simulink model "Waehrungsmodelle"  (R2014a)
settings: Solver=ode1  StartTime=0.0  StopTime=100  FixedStep=1  MaxStep=1  MinStep=1  RelTol=1e-3
(part 11 of 18)

== matlab function Waehrungsmodelle/Fließendes Währungssystem/Wechselkursberechnung/MATLAB Function ==
  data: GueterpreisAuslandInEigenwaehrung output; GueterpreisAusland input; Wechselkursfaktor output; GueterKonsumImInlandVomAusland input; GueterKonsumImAuslandVomInland input; GesamterGueterKonsumImAuslandVomInlandOut output; GesamterGueterKonsumImInlandVomAuslandOut output
function [GueterpreisAuslandInEigenwaehrung, Wechselkursfaktor, GesamterGueterKonsumImAuslandVomInlandOut, GesamterGueterKonsumImInlandVomAuslandOut] ...
        = Wechselkursberechnung(GueterpreisAusland, GueterKonsumImInlandVomAusland, GueterKonsumImAuslandVomInland)
%# Untermodul zur Berechnung eines realen Wechselkurses


% Aufsummierter Güterkonsum vom Ausland mit produzierten Gütern aus dem Inland
persistent GesamterGueterKonsumImAuslandVomInland;          
        
% Aufsummierter Güterkonsum vom Inland mit produzierten Gütern aus dem Ausland
persistent GesamterGueterKonsumImInlandVomAusland;    

% GesamterGueterKonsumImAuslandVomInland Initial
if isempty(GesamterGueterKonsumImAuslandVomInland)
   GesamterGueterKonsumImAuslandVomInland = 1;
end

% GueterKonsumImInlandVomAusland Initial
if isempty(GesamterGueterKonsumImInlandVomAusland)
   GesamterGueterKonsumImInlandVomAusland = 1;
end

GesamterGueterKonsumImAuslandVomInland = GesamterGueterKonsumImAuslandVomInland + GueterKonsumImAuslandVomInland;
GesamterGueterKonsumImInlandVomAusland = GesamterGueterKonsumImInlandVomAusland + GueterKonsumImInlandVomAusland;
   
% Berechnung eines realen Wechselkurses
Wechselkursfaktor =  GesamterGueterKonsumImInlandVomAusland / GesamterGueterKonsumImAuslandVomInland;

% Güterpreis der importierten Waren in Inländischer Währung
GueterpreisAuslandInEigenwaehrung = GueterpreisAusland * Wechselkursfaktor;

% Zustandswerte ausgeben
GesamterGueterKonsumImAuslandVomInlandOut = GesamterGueterKonsumImAuslandVomInland;
GesamterGueterKonsumImInlandVomAuslandOut = GesamterGueterKonsumImInlandVomAusland;

== matlab function Waehrungsmodelle/Währungssystem5/Haushalte/MATLAB Function ==
  data: Erwerbsfaehige input; GueterkonsumInland output; ArbeitsplaetzeDienstleistungen input; ArbeitsplaetzeUnternehmen input; NeueKreditvergabeInland input; KreditrueckzahlungInland input; GueterAngebotInland input; Arbeitslohn input; GueterpreisInland input; FinanzierungArbeitslosigkeit output; Spareinlagen output; KreditbedarfInland output; ArbeiterUnternehmen output; GueterVorratHaushalte output; GueterangebotsqualitaetOut output; Arbeitslosenquote output; GueterpreisAusland input; GueterkonsumAusland output; KreditbedarfAusland output; NeueKreditvergabeAusland input; KreditrueckzahlungAusland input; GueterAngebotAusland input; KreditZinssatzInland input; KreditZinssatzAusland input
function [GueterkonsumInland, FinanzierungArbeitslosigkeit, Spareinlagen, KreditbedarfInland, ...
              ArbeiterUnternehmen, GueterVorratHaushalte, GueterangebotsqualitaetOut, ...
              Arbeitslosenquote, GueterkonsumAusland, KreditbedarfAusland] = ...
    Haushalte(Erwerbsfaehige, ArbeitsplaetzeDienstleistungen, ArbeitsplaetzeUnternehmen, ...
            NeueKreditvergabeInland, KreditrueckzahlungInland, GueterAngebotInland, Arbeitslohn, ...
            GueterpreisInland, GueterpreisAusland, NeueKreditvergabeAusland, ...
            KreditrueckzahlungAusland, GueterAngebotAusland, KreditZinssatzInland, KreditZinssatzAusland)
 %# Submodul zur Berechnung der Abläufe bzgl. der Haushalte
 
% Es wird eine Gütereinheit pro Zeiteinheit und Erwerbsfaehiger
% verbraucht;
persistent GueterVorrat;

% Angebotsqualität der Güter [0 - 1]
% Werden weniger Güter angeboten als benötigt oder ist die Anzahl der 
% benötigten Güter nicht mehr bezahlbar sinkt die Qualität
persistent Gueterangebotsqualitaet;

    % Anfangsvorrat
    if isempty(GueterVorrat)
       GueterVorrat = 100;
    end 
    
    if isempty(Gueterangebotsqualitaet)
       Gueterangebotsqualitaet = 1;
    end     
    
    % Beschäftigte bei Öffentlichen Dienstleistungen bekommen 80 % vom
    % Lohnniveau der Unternehmen
    Dienstleistungslohnfaktor = 0.8;
    
    % Arbeitslose bekommen vom Staat 50% des Lohnnivaus
    Arbeitslosenlohnfaktor = 0.5;    
    
    % Maximale Vorratszeit
    MaximaleVorratszeit = 4;
    
    % Der maximale Vorrat gilt für 4 Zeiteinheiten
    MaximalerVorrat = Erwerbsfaehige * MaximaleVorratszeit; 
    
    
    % Gueterverbrauch pro Zeiteinheit
    GueterVorrat = GueterVorrat -  Erwerbsfaehige;    

    if GueterVorrat <= 0
         % Sind weniger Vorräte als fuer eine Zeiteinheit vorhanden, 
         % sinkt die Güterqualität
        Gueterangebotsqualitaet = Gueterangebotsqualitaet - 0.1;
        Gueterangebotsqualitaet = max(Gueterangebotsqualitaet, 0);
    else 
         % Sind mehr Vorräte als fuer eine Zeiteinheit vorhanden, 
         % steigt die Güterqualität        
        Gueterangebotsqualitaet = Gueterangebotsqualitaet + 0.1;
        Gueterangebotsqualitaet = min(Gueterangebotsqualitaet, 1);        
    end       
    
    GueterangebotsqualitaetOut = Gueterangebotsqualitaet;  
    
    % Es können maximal die vergleibenden Erwerbsfähigen oder der
    % notwendige Arbeiterbedarf eingesetzt werden
    ArbeiterUnternehmen = Erwerbsfaehige - ArbeitsplaetzeDienstleistungen;
    
    % die Arbeitslosen sind alle Erwerbsfähigen, welche keinen Arbeitsplatz
    % haben
    Arbeitslose = Erwerbsfaehige - (ArbeitsplaetzeUnternehmen + ArbeitsplaetzeDienstleistungen );
    % Arbeitslosenquote [0 - 1]
    % Auf Grund von Rundungen kann die Arbeitslosenquote min. 0 sein.
    Arbeitslosenquote = max(0, Arbeitslose / Erwerbsfaehige);
    
   
    
    % Einkommensberechnung für die Arbeitsplätze bei Unternehmen
    EinkommenUnternehmen = ArbeitsplaetzeUnternehmen * Arbeitslohn ;
    
    % Einkommensberechnung für die Arbeitsplätze bei Öffentlichen Dienstleistungen
    EinkommenDienstleistungen = ArbeitsplaetzeDienstleistungen * Arbeitslohn * Dienstleistungslohnfaktor;
    
    % Finanzierungsbedarf fuer Arbeitslosigkeit
    EinkommenArbeitslosigkeit = Arbeitslose * Arbeitslohn * Arbeitslosenlohnfaktor;
    FinanzierungArbeitslosigkeit = EinkommenArbeitslosigkeit;
    
    % Berechnung des Gesamteinkommens
    Gesamteinkommen = EinkommenUnternehmen + EinkommenDienstleistungen + EinkommenArbeitslosigkeit;           
        
    % Genehmigung der letzten Kreditanfrage
    Gesamteinkommen = Gesamteinkommen + NeueKreditvergabeInland + NeueKreditvergabeAusland;   
    
    % Rückzahlung der offenen Kreditrate
    Gesamteinkommen = Gesamteinkommen - KreditrueckzahlungInland - KreditrueckzahlungAusland;    
    
    % Prüfen welche Güter die günstigeren sind (Inlandsgüter oder
    % Auslandsgüter)
    if GueterpreisInland <= GueterpreisAusland
        % Wenn die Güter im Inland günstiger sind
        
        % Güter nachkaufen solange das Geld reicht oder das Vorratsmaximum erreicht
        % wurde, in Abhängigkeit des Güterangebots
        MoeglicheGueternachfrage = floor(Gesamteinkommen / GueterpreisInland);      
        % Die kleinste Gueternachfrage ist immer 50% des normalen
        % Verbrauchs der Güter
        GueterkonsumInland = max(0, min(MoeglicheGueternachfrage, GueterAngebotInland));

        % Wenn genug Güter auf Vorrat Komsum auf 50% senken
        if GueterVorrat > MaximalerVorrat
            GueterkonsumInland = GueterkonsumInland / 2;    
        end

        GueterVorrat = GueterVorrat + GueterkonsumInland;
        UebrigesGueterangebot = GueterAngebotInland - GueterkonsumInland;
        UebrigesEinkommen = Gesamteinkommen - (GueterkonsumInland * GueterpreisInland);  

        % Wenn noch Geld übrig ist und genug Geld vorhanden im Ausland die
        % Güter kaufen
        if GueterVorrat < MaximalerVorrat && UebrigesEinkommen > 0
            % Güter nachkaufen solange das Geld reicht oder das Vorratsmaximum erreicht
            % wurde, in Abhängigkeit des Güterangebots
            MoeglicheGueternachfrageAusland = floor(UebrigesEinkommen / GueterpreisAusland);              
            GueterkonsumAusland = max(0, min(min(MoeglicheGueternachfrageAusland, GueterAngebotAusland), MaximalerVorrat-GueterVorrat));           
            
            GueterVorrat = GueterVorrat + GueterkonsumAusland;
            UebrigesEinkommen = UebrigesEinkommen - (GueterkonsumAusland * GueterpreisAusland);                  
        else
            GueterkonsumAusland = 0;
        end        
    else
        % Wenn die Güter im Ausland günstiger sind
        
        % Güter nachkaufen solange das Geld reicht oder das Vorratsmaximum erreicht
        % wurde, in Abhängigkeit des Güterangebots
        % Es können maximal 50% der Güter aus dem Ausland gekauft werden
        MoeglicheGueternachfrage = min(0, min(Erwerbsfaehige/2, floor(Gesamteinkommen / GueterpreisAusland)));    

        GueterkonsumAusland = max(0, min(MoeglicheGueternachfrage, GueterAngebotAusland));

        % Wenn genug Güter auf Vorrat Komsum auf 50% senken
        if GueterVorrat > MaximalerVorrat
            GueterkonsumAusland = GueterkonsumAusland / 2;    
        end

        GueterVorrat = GueterVorrat + GueterkonsumAusland;

        UebrigesEinkommen = Gesamteinkommen - (GueterkonsumAusland * GueterpreisAusland);  

        % Wenn noch Geld übrig ist und genug Geld vorhanden im Ausland die
        % Güter kaufen
        if GueterVorrat < MaximalerVorrat && UebrigesEinkommen > 0
            % Güter nachkaufen solange das Geld reicht oder das Vorratsmaximum erreicht
            % wurde, in Abhängigkeit des Güterangebots
            MoeglicheGueternachfrageInland = floor(UebrigesEinkommen / GueterpreisInland);              
            GueterkonsumInland = max(0, min(MoeglicheGueternachfrageInland, GueterAngebotInland));                       
            GueterkonsumInland = GueterkonsumInland * min(0, 1.5 - GueterVorrat / MaximalerVorrat);
            
            GueterVorrat = GueterVorrat + GueterkonsumInland;
            UebrigesGueterangebot = GueterAngebotInland - GueterkonsumInland;
            UebrigesEinkommen = UebrigesEinkommen - (GueterkonsumInland * GueterpreisInland);                  
        else
            GueterkonsumInland = 0;
            UebrigesGueterangebot = 0;
        end            
    end   
    
    
    % Prüfung ob ein Kredit notwendig ist, da noch zu wenig Güter gekauft
    % wurden und Güter vorhanden sind
    if GueterVorrat < Erwerbsfaehige *2 && UebrigesGueterangebot > 0
        % Berechnung der notwendigen Güter bis zur nächsten Zeiteinheit
        BenoetigteGueter = Erwerbsfaehige;                
                        
        % Berechnung des Kreditbedarfs
        Kreditbedarf = BenoetigteGueter * GueterpreisInland;  
        % Kreditbedarf auf In- und Ausland aufteilen
        % Der Kredit mit dem geringeren Zinssatz wird bevorzugt und 70%
        % verwendet. Der teurere Kredit wird mit 30% verwendet.
        if KreditZinssatzInland <= KreditZinssatzAusland
            KreditbedarfInland = Kreditbedarf * 0.7;
            KreditbedarfAusland = Kreditbedarf * 0.3;
        else
            KreditbedarfAusland = Kreditbedarf * 0.7;
            KreditbedarfInland = Kreditbedarf * 0.3;        
        end        
    else
        % Kein Kreditbedarf
        KreditbedarfInland = 0;        
        KreditbedarfAusland = 0;  
    end
    
    % Übriges Geld sparen
    Spareinlagen = UebrigesEinkommen;
    
    GueterVorratHaushalte = GueterVorrat;

== matlab function Waehrungsmodelle/Vollgeld Währungssystem/Wechselkursberechnung/MATLAB Function ==
  data: GueterpreisAuslandInEigenwaehrung output; GueterpreisAusland input; Wechselkursfaktor output; GueterKonsumImInlandVomAusland input; GueterKonsumImAuslandVomInland input; GesamterGueterKonsumImAuslandVomInlandOut output; GesamterGueterKonsumImInlandVomAuslandOut output
function [GueterpreisAuslandInEigenwaehrung, Wechselkursfaktor, GesamterGueterKonsumImAuslandVomInlandOut, GesamterGueterKonsumImInlandVomAuslandOut] ...
        = Wechselkursberechnung(GueterpreisAusland, GueterKonsumImInlandVomAusland, GueterKonsumImAuslandVomInland)
%# Untermodul zur Berechnung eines realen Wechselkurses


% Aufsummierter Güterkonsum vom Ausland mit produzierten Gütern aus dem Inland
persistent GesamterGueterKonsumImAuslandVomInland;          
        
% Aufsummierter Güterkonsum vom Inland mit produzierten Gütern aus dem Ausland
persistent GesamterGueterKonsumImInlandVomAusland;    

% GesamterGueterKonsumImAuslandVomInland Initial
if isempty(GesamterGueterKonsumImAuslandVomInland)
   GesamterGueterKonsumImAuslandVomInland = 1;
end

% GueterKonsumImInlandVomAusland Initial
if isempty(GesamterGueterKonsumImInlandVomAusland)
   GesamterGueterKonsumImInlandVomAusland = 1;
end

GesamterGueterKonsumImAuslandVomInland = GesamterGueterKonsumImAuslandVomInland + GueterKonsumImAuslandVomInland;
GesamterGueterKonsumImInlandVomAusland = GesamterGueterKonsumImInlandVomAusland + GueterKonsumImInlandVomAusland;
   
% Berechnung eines realen Wechselkurses
Wechselkursfaktor =  GesamterGueterKonsumImInlandVomAusland / GesamterGueterKonsumImAuslandVomInland;

% Güterpreis der importierten Waren in Inländischer Währung
GueterpreisAuslandInEigenwaehrung = GueterpreisAusland * Wechselkursfaktor;

% Zustandswerte ausgeben
GesamterGueterKonsumImAuslandVomInlandOut = GesamterGueterKonsumImAuslandVomInland;
GesamterGueterKonsumImInlandVomAuslandOut = GesamterGueterKonsumImInlandVomAusland;

== matlab function Waehrungsmodelle/Währungssystem3/Haushalte/MATLAB Function ==
  data: Erwerbsfaehige input; GueterkonsumInland output; ArbeitsplaetzeDienstleistungen input; ArbeitsplaetzeUnternehmen input; NeueKreditvergabeInland input; KreditrueckzahlungInland input; GueterAngebotInland input; Arbeitslohn input; GueterpreisInland input; FinanzierungArbeitslosigkeit output; Spareinlagen output; KreditbedarfInland output; ArbeiterUnternehmen output; GueterVorratHaushalte output; GueterangebotsqualitaetOut output; Arbeitslosenquote output; GueterpreisAusland input; GueterkonsumAusland output; KreditbedarfAusland output; NeueKreditvergabeAusland input; KreditrueckzahlungAusland input; GueterAngebotAusland input; KreditZinssatzInland input; KreditZinssatzAusland input
function [GueterkonsumInland, FinanzierungArbeitslosigkeit, Spareinlagen, KreditbedarfInland, ...
              ArbeiterUnternehmen, GueterVorratHaushalte, GueterangebotsqualitaetOut, ...
              Arbeitslosenquote, GueterkonsumAusland, KreditbedarfAusland] = ...
    Haushalte(Erwerbsfaehige, ArbeitsplaetzeDienstleistungen, ArbeitsplaetzeUnternehmen, ...
            NeueKreditvergabeInland, KreditrueckzahlungInland, GueterAngebotInland, Arbeitslohn, ...
            GueterpreisInland, GueterpreisAusland, NeueKreditvergabeAusland, ...
            KreditrueckzahlungAusland, GueterAngebotAusland, KreditZinssatzInland, KreditZinssatzAusland)
 %# Submodul zur Berechnung der Abläufe bzgl. der Haushalte
 
% Es wird eine Gütereinheit pro Zeiteinheit und Erwerbsfaehiger
% verbraucht;
persistent GueterVorrat;

% Angebotsqualität der Güter [0 - 1]
% Werden weniger Güter angeboten als benötigt oder ist die Anzahl der 
% benötigten Güter nicht mehr bezahlbar sinkt die Qualität
persistent Gueterangebotsqualitaet;

    % Anfangsvorrat
    if isempty(GueterVorrat)
       GueterVorrat = 100;
    end 
    
    if isempty(Gueterangebotsqualitaet)
       Gueterangebotsqualitaet = 1;
    end     
    
    % Beschäftigte bei Öffentlichen Dienstleistungen bekommen 80 % vom
    % Lohnniveau der Unternehmen
    Dienstleistungslohnfaktor = 0.8;
    
    % Arbeitslose bekommen vom Staat 50% des Lohnnivaus
    Arbeitslosenlohnfaktor = 0.5;    
    
    % Maximale Vorratszeit
    MaximaleVorratszeit = 4;
    
    % Der maximale Vorrat gilt für 4 Zeiteinheiten
    MaximalerVorrat = Erwerbsfaehige * MaximaleVorratszeit; 
    
    
    % Gueterverbrauch pro Zeiteinheit
    GueterVorrat = GueterVorrat -  Erwerbsfaehige;    

    if GueterVorrat <= 0
         % Sind weniger Vorräte als fuer eine Zeiteinheit vorhanden, 
         % sinkt die Güterqualität
        Gueterangebotsqualitaet = Gueterangebotsqualitaet - 0.1;
        Gueterangebotsqualitaet = max(Gueterangebotsqualitaet, 0);
    else 
         % Sind mehr Vorräte als fuer eine Zeiteinheit vorhanden, 
         % steigt die Güterqualität        
        Gueterangebotsqualitaet = Gueterangebotsqualitaet + 0.1;
        Gueterangebotsqualitaet = min(Gueterangebotsqualitaet, 1);        
    end       
    
    GueterangebotsqualitaetOut = Gueterangebotsqualitaet;  
    
    % Es können maximal die vergleibenden Erwerbsfähigen oder der
    % notwendige Arbeiterbedarf eingesetzt werden
    ArbeiterUnternehmen = Erwerbsfaehige - ArbeitsplaetzeDienstleistungen;
    
    % die Arbeitslosen sind alle Erwerbsfähigen, welche keinen Arbeitsplatz
    % haben
    Arbeitslose = Erwerbsfaehige - (ArbeitsplaetzeUnternehmen + ArbeitsplaetzeDienstleistungen );
    % Arbeitslosenquote [0 - 1]
    % Auf Grund von Rundungen kann die Arbeitslosenquote min. 0 sein.
    Arbeitslosenquote = max(0, Arbeitslose / Erwerbsfaehige);
    
   
    
    % Einkommensberechnung für die Arbeitsplätze bei Unternehmen
    EinkommenUnternehmen = ArbeitsplaetzeUnternehmen * Arbeitslohn ;
    
    % Einkommensberechnung für die Arbeitsplätze bei Öffentlichen Dienstleistungen
    EinkommenDienstleistungen = ArbeitsplaetzeDienstleistungen * Arbeitslohn * Dienstleistungslohnfaktor;
    
    % Finanzierungsbedarf fuer Arbeitslosigkeit
    EinkommenArbeitslosigkeit = Arbeitslose * Arbeitslohn * Arbeitslosenlohnfaktor;
    FinanzierungArbeitslosigkeit = EinkommenArbeitslosigkeit;
    
    % Berechnung des Gesamteinkommens
    Gesamteinkommen = EinkommenUnternehmen + EinkommenDienstleistungen + EinkommenArbeitslosigkeit;           
        
    % Genehmigung der letzten Kreditanfrage
    Gesamteinkommen = Gesamteinkommen + NeueKreditvergabeInland + NeueKreditvergabeAusland;   
    
    % Rückzahlung der offenen Kreditrate
    Gesamteinkommen = Gesamteinkommen - KreditrueckzahlungInland - KreditrueckzahlungAusland;    
    
    % Prüfen welche Güter die günstigeren sind (Inlandsgüter oder
    % Auslandsgüter)
    if GueterpreisInland <= GueterpreisAusland
        % Wenn die Güter im Inland günstiger sind
        
        % Güter nachkaufen solange das Geld reicht oder das Vorratsmaximum erreicht
        % wurde, in Abhängigkeit des Güterangebots
        MoeglicheGueternachfrage = floor(Gesamteinkommen / GueterpreisInland);      
        % Die kleinste Gueternachfrage ist immer 50% des normalen
        % Verbrauchs der Güter
        GueterkonsumInland = max(0, min(MoeglicheGueternachfrage, GueterAngebotInland));

        % Wenn genug Güter auf Vorrat Komsum auf 50% senken
        if GueterVorrat > MaximalerVorrat
            GueterkonsumInland = GueterkonsumInland / 2;    
        end

        GueterVorrat = GueterVorrat + GueterkonsumInland;
        UebrigesGueterangebot = GueterAngebotInland - GueterkonsumInland;
        UebrigesEinkommen = Gesamteinkommen - (GueterkonsumInland * GueterpreisInland);  

        % Wenn noch Geld übrig ist und genug Geld vorhanden im Ausland die
        % Güter kaufen
        if GueterVorrat < MaximalerVorrat && UebrigesEinkommen > 0
            % Güter nachkaufen solange das Geld reicht oder das Vorratsmaximum erreicht
            % wurde, in Abhängigkeit des Güterangebots
            MoeglicheGueternachfrageAusland = floor(UebrigesEinkommen / GueterpreisAusland);              
            GueterkonsumAusland = max(0, min(min(MoeglicheGueternachfrageAusland, GueterAngebotAusland), MaximalerVorrat-GueterVorrat));           
            
            GueterVorrat = GueterVorrat + GueterkonsumAusland;
            UebrigesEinkommen = UebrigesEinkommen - (GueterkonsumAusland * GueterpreisAusland);                  
        else
            GueterkonsumAusland = 0;
        end        
    else
        % Wenn die Güter im Ausland günstiger sind
        
        % Güter nachkaufen solange das Geld reicht oder das Vorratsmaximum erreicht
        % wurde, in Abhängigkeit des Güterangebots
        % Es können maximal 50% der Güter aus dem Ausland gekauft werden
        MoeglicheGueternachfrage = min(0, min(Erwerbsfaehige/2, floor(Gesamteinkommen / GueterpreisAusland)));    

        GueterkonsumAusland = max(0, min(MoeglicheGueternachfrage, GueterAngebotAusland));

        % Wenn genug Güter auf Vorrat Komsum auf 50% senken
        if GueterVorrat > MaximalerVorrat
            GueterkonsumAusland = GueterkonsumAusland / 2;    
        end

        GueterVorrat = GueterVorrat + GueterkonsumAusland;

        UebrigesEinkommen = Gesamteinkommen - (GueterkonsumAusland * GueterpreisAusland);  

        % Wenn noch Geld übrig ist und genug Geld vorhanden im Ausland die
        % Güter kaufen
        if GueterVorrat < MaximalerVorrat && UebrigesEinkommen > 0
            % Güter nachkaufen solange das Geld reicht oder das Vorratsmaximum erreicht
            % wurde, in Abhängigkeit des Güterangebots
            MoeglicheGueternachfrageInland = floor(UebrigesEinkommen / GueterpreisInland);              
            GueterkonsumInland = max(0, min(MoeglicheGueternachfrageInland, GueterAngebotInland));                       
            GueterkonsumInland = GueterkonsumInland * min(0, 1.5 - GueterVorrat / MaximalerVorrat);
            
            GueterVorrat = GueterVorrat + GueterkonsumInland;
            UebrigesGueterangebot = GueterAngebotInland - GueterkonsumInland;
            UebrigesEinkommen = UebrigesEinkommen - (GueterkonsumInland * GueterpreisInland);                  
        else
            GueterkonsumInland = 0;
            UebrigesGueterangebot = 0;
        end            
    end   
    
    
    % Prüfung ob ein Kredit notwendig ist, da noch zu wenig Güter gekauft
    % wurden und Güter vorhanden sind
    if GueterVorrat < Erwerbsfaehige *2 && UebrigesGueterangebot > 0
        % Berechnung der notwendigen Güter bis zur nächsten Zeiteinheit
        BenoetigteGueter = Erwerbsfaehige;                
                        
        % Berechnung des Kreditbedarfs
        Kreditbedarf = BenoetigteGueter * GueterpreisInland;  
        % Kreditbedarf auf In- und Ausland aufteilen
        % Der Kredit mit dem geringeren Zinssatz wird bevorzugt und 70%
        % verwendet. Der teurere Kredit wird mit 30% verwendet.
        if KreditZinssatzInland <= KreditZinssatzAusland
            KreditbedarfInland = Kreditbedarf * 0.7;
            KreditbedarfAusland = Kreditbedarf * 0.3;
        else
            KreditbedarfAusland = Kreditbedarf * 0.7;
            KreditbedarfInland = Kreditbedarf * 0.3;        
        end        
    else
        % Kein Kreditbedarf
        KreditbedarfInland = 0;        
        KreditbedarfAusland = 0;  
    end
    
    % Übriges Geld sparen
    Spareinlagen = UebrigesEinkommen;
    
    GueterVorratHaushalte = GueterVorrat;

== matlab function Waehrungsmodelle/Gedecktes Währungssystem/Öffentliche Dienstleistungen/MATLAB Function ==
  data: Finanzierung input; ArbeitsplaetzeDienstleistung output; Erwerbsfaehige input; Arbeitslohn input; Dienstleistungsqualitaet output
function [ArbeitsplaetzeDienstleistung, Dienstleistungsqualitaet] = OeffentlicheDienstleistungen(Finanzierung, Erwerbsfaehige, Arbeitslohn)
%# Submodul zur Berechnung das Öffentliche Dienstleistungsmodell

    persistent Arbeitsplaetze;

    % Anfangsarbeitsplätze
    if isempty(Arbeitsplaetze)
       Arbeitsplaetze = 20;
    end 

    % Da der Arbeitslohn ein Referenzlohn der privaten Unternehmen ist wird
    % dieser angepasst und um 20 % gesenkt
    LohnNiveauOeffentlicherDienst = 0.8;
    Arbeitslohn = Arbeitslohn * LohnNiveauOeffentlicherDienst;
    
    % Es können nicht mehr Arbeitsplätze wie Erwerbsfähige vorhanden sind
    % besetzt werden
    if Erwerbsfaehige < Arbeitsplaetze
        Arbeitsplaetze = Erwerbsfaehige;
    end

    % Existiert nicht genug Geld für die öffentlichen Dientleistungen
    % werden die Arbeitsplätze an die Finanzierung vom Staat angepasst.
    if (Finanzierung < Arbeitsplaetze * Arbeitslohn)
        Arbeitsplaetze = floor(Finanzierung / Arbeitslohn);        
    end          
       
    ArbeitsplaetzeDienstleistung = Arbeitsplaetze;
    
    % Berechnet Dienstleistungsqualitaet mit min:0.2 und max:1
    % indem die Arbeitsplätze der öffentlichen Dienstleistungen durch die
    % gesamten Erwerbstätigen geteilt werden und als Ausgleichfaktor mit drei
    % multipliziert wird. Somit ist es optimal wenn min. 1/3 aller
    % Erwerbsfähigen bei den öffentlichen Dienstleistungen arbeiten
    Dienstleistungsqualitaet = max(0.2, min(1, 3 * Arbeitsplaetze / Erwerbsfaehige));

== matlab function Waehrungsmodelle/Währungssystem6/Notenbank/MATLAB Function ==
  data: Gesamtkredite input; LeitzinsOut output; MindestreservesatzOut output; MaximaleNotenbankGeldmengeOut output; Arbeitslosenquote input; Inflation input; Wirtschaftswachtsum input
function [LeitzinsOut, MindestreservesatzOut, MaximaleNotenbankGeldmengeOut] = ...
    Notenbank(Gesamtkredite, Arbeitslosenquote, Inflation, Wirtschaftswachtsum)
%# Submodul zur Berechnung der Notenbankprozesse

% Leitzins der Notenbank => 0.03
persistent Leitzins;

% Mindestreservesatz => 0.01
persistent Mindestreservesatz;    

% Maximale Geldmenge, welche von der Notenbank vergeben werden kann
persistent MaximaleNotenbankGeldmenge;   

% festgelegter Geldmengenwachstum => 0.05
% Dieser Wert ist bei gedeckten Währungssystemen notwendig, da hiermit die
% Geldmenge mit dem Gesamtwert des Deckungswerts mitwachsen kann
Geldmengenwachstum = 0.05;

% gewünschte Inflation => 0.02
Inflationsziel = 0.02;

% Inflationstoleranz => 0.02
Inflationstoleranz = 0.02;

% Arbeitslosentoleranzquote => 0.08
Arbeitslosentoleranzquote = 0.08;

% Änderung des Leitzins
Leitzinsaenderung = 0;

    if isempty(Leitzins)
       Leitzins = 0.03;
    end  
    if isempty(Mindestreservesatz)
       Mindestreservesatz = 0.01;
    end  
    if isempty(MaximaleNotenbankGeldmenge)
       MaximaleNotenbankGeldmenge =  1000;
    end       
    
    % Pürfen, ob ein erlaubter Geldmengenwachstum sinnvoll ist
    if Gesamtkredite > MaximaleNotenbankGeldmenge * 0.9
        MaximaleNotenbankGeldmenge = MaximaleNotenbankGeldmenge * (1 + Geldmengenwachstum);
    end
    
    % Wenn das Wirtschaftswachtsum zu gering ist, wird der Leitzins gesenkt
    if Wirtschaftswachtsum < Leitzins
        Leitzinsaenderung = -0.001;
    else
        Leitzinsaenderung = 0.001;
    end
    
    % Wenn die Arbeitslosigkeit unter der Arbeitslosentoleranzquote ist, wird kann der Leitzins erhöht
    % sonst wird der Leitzins in Abhängigkeit der Arbeitslosenquote gesenkt
    Leitzinsaenderung = Leitzinsaenderung + max(-0.01,0.1 * (Arbeitslosentoleranzquote - Arbeitslosenquote) + 0.001); 
    
    % Inflation mit dem Leitzins an die Zielinflation anpassen
    Leitzinsaenderung = Leitzinsaenderung + 0.01 * (Inflation - (Inflationsziel + Inflationstoleranz));
        
    if Leitzins < 0.01 && Leitzinsaenderung < -0.001
        Leitzins = Leitzins - 0.001;
    else        
        Leitzins = Leitzins + Leitzinsaenderung;
    end
    
LeitzinsOut = Leitzins;
MindestreservesatzOut = Mindestreservesatz;
MaximaleNotenbankGeldmengeOut = MaximaleNotenbankGeldmenge;

== matlab function Waehrungsmodelle/Währungssystem6/Unternehmen/MATLAB Function ==
  data: Inflation output; Rohstoffbedarf output; ArbeitsplaetzeUnternehmen output; GueterangebotInland output; ArbeitslohnOut output; Erwerbsfaehige input; BenoetigterArbeitsbedarfUnternehmen output; GueterpreisOut output; NeueKreditvergabeUnternehmen input; KreditrueckzahlungUnternehmen input; SteuernUnternehmen output; RessourcenAbgabeSteuer output; KreditbedarfInland output; Rohstoffe input; GueterkonsumInland input; GueterkonsumAusland input; RessourcenAbgabeSteuersatz input; KreditZinssatzInland input; KreditZinssatzAusland input; Steuersatz input; KreditbedarfAusland output; TechnischeVerbesserungRationalitaetOut output; TechnischeVerbesserungRessourcenOut output; Wirtschaftswachstum output; GueterangebotAusland output; NeueKreditvergabeUnternehmenAusland input; KreditrueckzahlungUnternehmenAusland input
function [Inflation, Rohstoffbedarf, ArbeitsplaetzeUnternehmen, GueterangebotInland, ...
            ArbeitslohnOut, BenoetigterArbeitsbedarfUnternehmen, GueterpreisOut, ...
            SteuernUnternehmen, RessourcenAbgabeSteuer, KreditbedarfInland, KreditbedarfAusland,  ...
            TechnischeVerbesserungRationalitaetOut, TechnischeVerbesserungRessourcenOut, ...
            Wirtschaftswachstum, GueterangebotAusland] = ...
   Unternehmen(Erwerbsfaehige, NeueKreditvergabeUnternehmen, KreditrueckzahlungUnternehmen, ...
            Rohstoffe, GueterkonsumInland, GueterkonsumAusland, RessourcenAbgabeSteuersatz, ...
            KreditZinssatzInland, KreditZinssatzAusland, Steuersatz, ...
            NeueKreditvergabeUnternehmenAusland, KreditrueckzahlungUnternehmenAusland)
        %# Submodul zur Berechnung der Prozessabläufe in Beziehung mit den Unternehmen

% Arbeitslohn
persistent Arbeitslohn;          
        
% Geldbestand
persistent Geldbestand;  
        
% Rohstoffbestand
persistent Rohstoffbestand;   
        
% produzierter Güterbestand
persistent Gueterbestand;   

% Preis zu dem das produzierte Gut verkauft wird
persistent Gueterpreis;  

% technische Effizienzverbesserung bzgl. der Rationalisierung der Arbeiter
persistent TechnischeVerbesserungRationalitaet;   

% technische Effizienzverbesserung bzgl. der Ressourcenverwendung
persistent TechnischeVerbesserungRessourcen;

% Letzte Anzahl an Mitarbeitern
persistent LetzteArbeitsplaetzeUnternehmen;

% Umsatz / Einnahmen
persistent Einnahmen;

% alte Inflation
persistent InflationAlt;

% Geldbestand Initial
if isempty(Geldbestand)
   Geldbestand = 50;
end
% Arbeitslohn Initial
if isempty(Arbeitslohn)
   Arbeitslohn = 3.5;
end
% Rohstoffbestand Initial
if isempty(Rohstoffbestand)
   Rohstoffbestand = 50;
end
% Güterbestand Initial
if isempty(Gueterbestand)
   Gueterbestand = 50;
end 
% Güterpreis Initial
if isempty(Gueterpreis)
   Gueterpreis = 3;
end 
% technische Effizienzverbesserung Rationalisierung Initial
if isempty(TechnischeVerbesserungRessourcen)
   TechnischeVerbesserungRessourcen = 1;
end
% technische Effizienzverbesserung Ressourcenverwendung Initial
if isempty(TechnischeVerbesserungRationalitaet)
   TechnischeVerbesserungRationalitaet = 1;
end
% Umsatz / Einnahmen Initial
if isempty(Einnahmen)
   Einnahmen = 0;
end
if isempty(InflationAlt)
   InflationAlt = 0;
end
% Letzte Anzahl an Mitarbeitern
if isempty(LetzteArbeitsplaetzeUnternehmen)
   LetzteArbeitsplaetzeUnternehmen = 20;
end

% Steigerung der Effizienzen bei technischen Verbesserungen Rationalität
EffizienzsteigerungRationalitaet = 0.04;
% Steigerung der Effizienzen bei technischen Verbesserungen Ressourcen
EffizienzsteigerungRessourcen = 0.02;
% Kosten einer technischen Verbesserung
Verbesserungskosten = 20;
% Steigerung der Kosten bei technischen Verbesserungen
Verbesserungskostensteigerung = 0.2;
% Angestrebter Gewinn
AngestrebterGewinn = 0.1;
% Maximale Preissteierung
MaximalePreissteierung = 0.15;
% Speicherung des letzten Güterpreises
AlterGueterpreis = Gueterpreis;
% Speicherung der letzten Einnahmen
AlteEinnahmen = Einnahmen;
% Menge produzierter Güter pro Mitarbeiter
ProduzierteMengeProMitarbeiter = 1.2;
% Gehaltssteigerung bei Rationalisierung und Gewinn
Gehaltssteigerung = 0.05;
% angestrebter Gütervorrat
GewuenschterGuetervorrat = 200;
% angestrebter Geldbestand
GewuenschterGeldbestand = 200;
% Maximale Entlassungen in Prozent
MaximaleEntlassungsrate = 0.2;

    % vergebene Kredite
    Geldbestand = Geldbestand + NeueKreditvergabeUnternehmen + NeueKreditvergabeUnternehmenAusland;
    % Ratenzahlung der aktuelen Kredite
    Geldbestand = Geldbestand - KreditrueckzahlungUnternehmen + KreditrueckzahlungUnternehmenAusland;

    % Berechnung der Ressourcenangabe
    RessourcenAbgabeSteuer = max(0, RessourcenAbgabeSteuersatz) * Rohstoffe;
    Rohstoffbestand = Rohstoffbestand + Rohstoffe;
    
    % In- und Auslandskonsum summieren
    Gueterkonsum = GueterkonsumInland + GueterkonsumAusland;
    
    % Güterbestand nach den von abgenommene Güter der Haushalten bei 
    % der letzten Zeiteinheit 
    Gueterbestand = Gueterbestand - Gueterkonsum;
    
    % Berechnung der Einnahmen
    Einnahmen = Gueterkonsum * Gueterpreis;
    
    % Berechnung der zu produzierenden Gütermenge (mit 30% Reserve) wenn
    % der Bestand kleiner als 200% des Güterkonsums in einer Zeiteinheit
    % Dabei werden 50 Güter als Reserve in Bestand vorgehalten
    if Gueterbestand < Gueterkonsum * 2
        ProduzierndeGuetermenge = max(5, (1.3 * Gueterkonsum) - (Gueterbestand - GewuenschterGuetervorrat));  
    elseif Gueterbestand < GewuenschterGuetervorrat
        ProduzierndeGuetermenge = Gueterkonsum + (GewuenschterGuetervorrat - Gueterbestand);
    else
       ProduzierndeGuetermenge = max(5, Gueterkonsum / 2);      
    end
    
    % Produktiongüter pro Mitarbeiter in Abhängigkeit
    % der technischen Verbesserung (normal 2 Güter pro Mitarbeiter)
    ProduktionProMitarbeiter = (((1 + EffizienzsteigerungRationalitaet) ^ TechnischeVerbesserungRationalitaet) * ProduzierteMengeProMitarbeiter);
    
    % Ressourcen pro hergestelltes Gut in Abhängigkeit
    % der technischen Verbesserung (normal 1 Güter pro Ressource)    
    RessourcenProGut = (1 / (1 + EffizienzsteigerungRessourcen)) ^ TechnischeVerbesserungRessourcen;
    
    % Zur Berechnung der benötigten Arbeitskraft im nächsten Zeitabschnitt´
    BenoetigterArbeitsbedarfUnternehmen = floor(ProduzierndeGuetermenge / ProduktionProMitarbeiter) + 1;           
    
    % Berechnung der maximal erstellbaren Gütermenge
    MaximaleGueterherstellungErwerbstaetige = Erwerbsfaehige * ProduktionProMitarbeiter;
    MaximaleGueterherstellungRohstoffe = Rohstoffbestand / RessourcenProGut;    
    % Entweder ist die Herstellung durch die Nachfrage, den Arbeitskreaften
    % oder den Ressourcen beschränkt
    Gueterherstellung = min(ProduzierndeGuetermenge, min(MaximaleGueterherstellungErwerbstaetige, MaximaleGueterherstellungRohstoffe));
    Gueterherstellung = max(Gueterherstellung, 0);  
    
    % Berechnung der aktuellen Arbeitsplätze
    ArbeitsplaetzeUnternehmen = floor(Gueterherstellung / ProduktionProMitarbeiter)+1;
    
    % Berechnung der maximalen möglichen Entlassungen
    % Es können max. 20% der Mitarbeiter entlassen werden    
    if ArbeitsplaetzeUnternehmen < LetzteArbeitsplaetzeUnternehmen * (1-MaximaleEntlassungsrate)
        ArbeitsplaetzeUnternehmen = LetzteArbeitsplaetzeUnternehmen * (1-MaximaleEntlassungsrate);
        MaximaleGueterherstellungErwerbstaetige = ArbeitsplaetzeUnternehmen * ProduktionProMitarbeiter;
        Gueterherstellung = min(ProduzierndeGuetermenge, min(MaximaleGueterherstellungErwerbstaetige, MaximaleGueterherstellungRohstoffe));        
    end
    
    % Vergleich der Arbeitsnachfrage mit dem Arbeitsangebot
    ArbeitsangebotsNachfrageQuotient = ArbeitsplaetzeUnternehmen / Erwerbsfaehige;
    % Anpassung der Arbeitslöhne an das Angebot und die Nachfrage der
    % Arbeitsplaetze - max 3% Lohnsenkung oder Lohnsteigerung
    ArbeitsangebotsNachfrageQuotient= max(0.94,min(1.04,(ArbeitsangebotsNachfrageQuotient + 0.3)));
    Arbeitslohn = Arbeitslohn * ArbeitsangebotsNachfrageQuotient;
    
    % Berechnung der aktuell verbrauchten Ressourcen
    Rohstoffbestand = Rohstoffbestand - (floor(Gueterherstellung * RessourcenProGut)+1);
    
    % hergestellte Gütermenge
    Gueterbestand = Gueterbestand + Gueterherstellung;
    
    % Als Export-Angebot werden 30% der Güter vorgesehen
    GueterangebotAusland = Gueterbestand * 0.3;
    GueterangebotInland = Gueterbestand - GueterangebotAusland;          
    
    % Berechnung der Gehälter
    Gehaelter = ArbeitsplaetzeUnternehmen * Arbeitslohn;
    
    % Vorteil einer Investitionen-Rationalität berechnen
    InvestPruefungProduktionProMitarbeiter = (((1 + EffizienzsteigerungRationalitaet) ^ (TechnischeVerbesserungRationalitaet + 1)) * 2);
    InvestPruefungArbeitsplaetzeUnternehmen = floor(Gueterherstellung / InvestPruefungProduktionProMitarbeiter)+1;    
    InvesteinsparungRationalitaet = Arbeitslohn * (ArbeitsplaetzeUnternehmen - InvestPruefungArbeitsplaetzeUnternehmen);
    % Vorteil einer Investitionen-Ressourceneffizienz berechnen
    InvestPruefungRessourcenProGut = (1 / (1 + EffizienzsteigerungRessourcen)) ^ (TechnischeVerbesserungRessourcen + 1);
    InvestPruefungRessourcenbedarf = floor(Gueterherstellung * InvestPruefungRessourcenProGut)+1;    
    InvesteinsparungRessourcenbedarf = RessourcenAbgabeSteuersatz * ((Gueterherstellung * RessourcenProGut) - InvestPruefungRessourcenbedarf);    
    
    % Kosten für die nächste Investitionsstufe berechnen
    InvestkostenRationalitaet = Verbesserungskosten * (1 + Verbesserungskostensteigerung) ^ (TechnischeVerbesserungRationalitaet + 1);
    InvestkostenRessourcenEffizienz = Verbesserungskosten * (1 + Verbesserungskostensteigerung) ^ (TechnischeVerbesserungRessourcen + 1);
    
    % Prüfen, ob und welche Investition mehr Sinn macht
    % Das vorhandene Geld muss dabei doppelt so hoch sein, damit nicht mit
    % dem letzten Geld Investitionen durchgeführt werden
    Investition = 0;
    if (InvesteinsparungRationalitaet > InvesteinsparungRessourcenbedarf) && Geldbestand > InvestkostenRationalitaet*2 && InvesteinsparungRationalitaet > 0
        % Verbesserung Rationalität
        TechnischeVerbesserungRationalitaet = TechnischeVerbesserungRationalitaet + 1;
        Investition = InvestkostenRationalitaet;
        % Anstieg des Arbeitslohn auf Grund der Rationalitätsgewinne 
        Arbeitslohn = Arbeitslohn * (1 + Gehaltssteigerung);
    elseif Geldbestand > InvestkostenRessourcenEffizienz*2 && InvesteinsparungRessourcenbedarf > 0;
        % Verbesserung Ressourceneffizienz
        TechnischeVerbesserungRessourcen = TechnischeVerbesserungRessourcen + 1;
        Investition = InvestkostenRessourcenEffizienz;
    end
    
    % Ausgaben berechnen
    Ausgaben = RessourcenAbgabeSteuer + Gehaelter;
    
    % Der Preis der produzierten Warten richtet sich NICHT nach der Nachfrage 
    % und dem Angebot, sondern nach den Herrstellungskosten und dem 
    % angestrebten Gewinn. Welches ist der niedrigste Preis, damit das 
    % Unternehmen den angestrebten Gewinn erwirtschaftet und Investieren
    % kann
    Herstellkosten = Ausgaben / Gueterherstellung;
    % Es gibt eine maximale Preisteigerung welche durchgesetzt werden kann
    MaximalerGueterpreis = (1 + MaximalePreissteierung) * Gueterpreis;
    Gueterpreis = min(MaximalerGueterpreis, Herstellkosten * (1 + AngestrebterGewinn));   
    
    % Berechnung der Inflation
    Inflation = (InflationAlt + (Gueterpreis / AlterGueterpreis) - 1) / 2;
    InflationAlt = Inflation;
                
    % Gewinnberechnung
    Gewinn = Einnahmen - Ausgaben;            
    
    if Gewinn > 0
        % Anstieg des Arbeitslohn auf Grund der Gewinnsteigerung               
        Arbeitslohn = Arbeitslohn * (1 + Gehaltssteigerung);  
        
        % Steuerberechnung vom Gewinn
        SteuernUnternehmen = Gewinn * Steuersatz;
    else
        SteuernUnternehmen = 0;
    end

    Geldbestand = Geldbestand + Gewinn - (SteuernUnternehmen + Investition);
       
    % Wenn notwendig, neuen Kredit beantragen
    if Geldbestand < GewuenschterGeldbestand                
        % Kreditbedarf berechnen
        Kreditbedarf = GewuenschterGeldbestand - Geldbestand;
    else 
        Kreditbedarf = 0;
    end         
    
    % Kreditbedarf auf In- und Ausland aufteilen
    % Der Kredit mit dem geringeren Zinssatz wird bevorzugt und 70%
    % verwendet. Der teurere Kredit wird mit 30% verwendet.
    if KreditZinssatzInland <= KreditZinssatzAusland
        KreditbedarfInland = Kreditbedarf * 0.7;
        KreditbedarfAusland = Kreditbedarf * 0.3;
    else
        KreditbedarfAusland = Kreditbedarf * 0.7;
        KreditbedarfInland = Kreditbedarf * 0.3;        
    end

    % Berechnung der benötigten Ressourcen im nächsten Zeitabschnitt    
    Rohstoffbedarf = max(0, floor(Gueterherstellung * RessourcenProGut) + GewuenschterGuetervorrat - Rohstoffbestand);            
    
    % Auf Grund der Angebots-/Nachfragesituation kann der Güterpreis nicht
    % unter dem Arbeitslohn sein
    Gueterpreis = min(Gueterpreis, Arbeitslohn);
    % Wenn kein Konsum stattgefunden hat sinkt der Preis
    if GueterkonsumInland == 0
        Gueterpreis = Gueterpreis * (1-MaximalePreissteierung);
    end
    
    
    Wirtschaftswachstum = (Einnahmen / AlteEinnahmen) - 1;
    
    ArbeitslohnOut = Arbeitslohn;
    GueterpreisOut = Gueterpreis;
    TechnischeVerbesserungRationalitaetOut = TechnischeVerbesserungRationalitaet;
    TechnischeVerbesserungRessourcenOut = TechnischeVerbesserungRessourcen;
    LetzteArbeitsplaetzeUnternehmen = ArbeitsplaetzeUnternehmen;

== system Waehrungsmodelle/Vollgeld Währungssystem/Wechselkursberechnung ==
  Güterpreis Ausland : Inport
  Güterkonsum im Inland von Gütern vom Ausland : Inport  Port=2
  Güterkonsum im Ausland von Gütern im Inland : Inport  Port=3
  MATLAB Function : MATLAB Function  TreatAsAtomicUnit=on
  Güterpreis Ausland in Eigenwährung : Outport
  Wechselkursfaktor : Outport  Port=2
  Gesamter Güterkonsum im Ausland von Gütern im Inland : Outport  Port=3
  Gesamter Güterkonsum im Inland von Gütern vom Ausland : Outport  Port=4
  wires:
  Güterpreis Ausland/1 -> MATLAB Function/1(GueterpreisAusland)
  Güterkonsum im Inland von Gütern vom Ausland/1 -> MATLAB Function/2(GueterKonsumImInlandVomAusland)
  Güterkonsum im Ausland von Gütern im Inland/1 -> MATLAB Function/3(GueterKonsumImAuslandVomInland)
  MATLAB Function/1(GueterpreisAuslandInEigenwaehrung) -> Güterpreis Ausland in Eigenwährung/1
  MATLAB Function/2(Wechselkursfaktor) -> Wechselkursfaktor/1
  MATLAB Function/3(GesamterGueterKonsumImAuslandVomInlandOut) -> Gesamter Güterkonsum im Ausland von Gütern im Inland/1
  MATLAB Function/4(GesamterGueterKonsumImInlandVomAuslandOut) -> Gesamter Güterkonsum im Inland von Gütern vom Ausland/1

== system Waehrungsmodelle/Vollgeld Währungssystem/Öffentliche Dienstleistungen ==
  Finanzierung : Inport
  Erwerbsfähige : Inport  Port=2
  Arbeitslohn : Inport  Port=3
  MATLAB Function : MATLAB Function  TreatAsAtomicUnit=on
  Arbeitsplätze Dienstleistung : Outport
  Dienstleistungsqualität : Outport  Port=2
  wires:
  Arbeitslohn/1 -> MATLAB Function/3(Arbeitslohn)
  Erwerbsfähige/1 -> MATLAB Function/2(Erwerbsfaehige)
  Finanzierung/1 -> MATLAB Function/1(Finanzierung)
  MATLAB Function/1(ArbeitsplaetzeDienstleistung) -> Arbeitsplätze Dienstleistung/1
  MATLAB Function/2(Dienstleistungsqualitaet) -> Dienstleistungsqualität/1

== system Waehrungsmodelle/Währungssystem1/Banken ==
  Einlangenänderung der Haushalte : Inport
  Kreditbedarf der Haushalte : Inport  Port=2
  Kreditbedarf der Unternehmen : Inport  Port=3
  Kreditbedarf der Haushalte im Ausland : Inport  Port=4
  Kreditbedarf der Unternehmen im Ausland : Inport  Port=5
  Kreditbedarf des Staates : Inport  Port=6
  Steuersatz : Inport  Port=7
  Leitzins der Notenbank : Inport  Port=8
  Mindestreservesatz der Notenbank : Inport  Port=9
  Maximale Geldmenge der Notebank : Inport  Port=10
  MATLAB Function : MATLAB Function  TreatAsAtomicUnit=on
  Kontostand der Haushalte : Outport
  Kredite der Haushalte : Outport  Port=2
  Kredite der Unternehmen : Outport  Port=3
  Kredite des Staates : Outport  Port=4
  Neue Kreditvergabe Haushalte : Outport  Port=5
  Neue Kreditvergabe Unternehmen : Outport  Port=6
  Neue Kreditvergabe Staat : Outport  Port=7
  Bankgewinn nach Steuern : Outport  Port=8
  Banksteuern : Outport  Port=9
  Bankkontostand : Outport  Port=10
  Bankenzinssatz : Outport  Port=11
  Kreditrückzahlung Staat : Outport  Port=12
  Kreditrückzahlung Haushalte : Outport  Port=13
  Kreditrückzahlung Unternehmen : Outport  Port=14
  Kredite der Unternehmen im Ausland : Outport  Port=15
  Kreditrückzahlung der Unternehmen im Ausland : Outport  Port=16
  Kreditvergabe der Unternehmen im Ausland : Outport  Port=17
  Kredite der Haushalte im Ausland : Outport  Port=18
  Kreditrückzahlung der Haushalte im Ausland : Outport  Port=19
  Kreditvergabe der Haushalte im Ausland : Outport  Port=20
  wires:
  MATLAB Function/1(KontoHaushalteOut) -> Kontostand der Haushalte/1
  MATLAB Function/2(KrediteHaushalteOut) -> Kredite der Haushalte/1
  MATLAB Function/3(KrediteUnternehmenOut) -> Kredite der Unternehmen/1
  MATLAB Function/4(KrediteStaatOut) -> Kredite des Staates/1
  MATLAB Function/5(KreditvergabeHaushalte) -> Neue Kreditvergabe Haushalte/1
  MATLAB Function/6(KreditvergabeUnternehmen) -> Neue Kreditvergabe Unternehmen/1
  MATLAB Function/7(KreditvergabeStaat) -> Neue Kreditvergabe Staat/1
  MATLAB Function/11(BankgewinnNachSteuern) -> Bankgewinn nach Steuern/1
  MATLAB Function/10(KreditrueckzahlungStaat) -> Kreditrückzahlung Staat/1
  MATLAB Function/9(KreditrueckzahlungUnternehmen) -> Kreditrückzahlung Unternehmen/1
  MATLAB Function/8(KreditrueckzahlungHaushalte) -> Kreditrückzahlung Haushalte/1
  MATLAB Function/14(Bankenzinssatz) -> Bankenzinssatz/1
  MATLAB Function/13(BankKontostand) -> Bankkontostand/1
  MATLAB Function/12(BankenSteuern) -> Banksteuern/1
  MATLAB Function/15(KrediteUnternehmenAuslandOut) -> Kredite der Unternehmen im Ausland/1
  MATLAB Function/16(KreditrueckzahlungUnternehmenAusland) -> Kreditrückzahlung der Unternehmen im Ausland/1
  MATLAB Function/17(KreditvergabeUnternehmenAusland) -> Kreditvergabe der Unternehmen im Ausland/1
  MATLAB Function/18(KrediteHaushalteAuslandOut) -> Kredite der Haushalte im Ausland/1
  MATLAB Function/20(KreditvergabeHaushalteAusland) -> Kreditvergabe der Haushalte im Ausland/1
  MATLAB Function/19(KreditrueckzahlungHaushalteAusland) -> Kreditrückzahlung der Haushalte im Ausland/1
  Einlangenänderung der Haushalte/1 -> MATLAB Function/1(EinlagenAenderungHaushalte)
  Kreditbedarf der Haushalte/1 -> MATLAB Function/2(KreditbedarfHaushalte)
  Kreditbedarf der Unternehmen/1 -> MATLAB Function/3(KreditbedarfUnternehmen)
  Kreditbedarf der Haushalte im Ausland/1 -> MATLAB Function/4(KreditbedarfHaushalteAusland)
  Kreditbedarf der Unternehmen im Ausland/1 -> MATLAB Function/5(KreditbedarfUnternehmenAusland)
  Kreditbedarf des Staates/1 -> MATLAB Function/6(KreditbedarfStaat)
  Steuersatz/1 -> MATLAB Function/7(Steuersatz)
  Leitzins der Notenbank/1 -> MATLAB Function/8(Leitzins)
  Mindestreservesatz der Notenbank/1 -> MATLAB Function/9(Mindestreservesatz)
  Maximale Geldmenge der Notebank/1 -> MATLAB Function/10(MaximaleNotenbankGeldmenge)

== system Waehrungsmodelle/Währungssystem1/Haushalte ==
  Erwerbsfähige : Inport
  Arbeitsplätze Dienstleistungen : Inport  Port=2
  Güterangebot Inland : Inport  Port=3
  Arbeitslohn : Inport  Port=4
  Güterpreis Inland : Inport  Port=5
  Neue Kreditvergabe Inland : Inport  Port=6
  Arbeitsplätze Unternehmen : Inport  Port=7
  Kreditrückzahlung Ausland : Inport  Port=8
  Güterpreis Ausland : Inport  Port=9
  Neue Kreditvergabe Ausland : Inport  Port=10
  Kreditrückzahlung Inland : Inport  Port=11
  Güterangebot Ausland : Inport  Port=12
  Kreditzinssatz Inland : Inport  Port=13
  Kreditzinssatz Ausland : Inport  Port=14
  MATLAB Function : MATLAB Function  TreatAsAtomicUnit=on
  Güterkonsum Inland : Outport
  Finanzbedarf Arbeitslosigkeit : Outport  Port=2
  Spareinlagen : Outport  Port=3
  Kreditbedarf Inland : Outport  Port=4
  Arbeiter Unternehmen : Outport  Port=5
  Gütervorrat der Haushalte : Outport  Port=6
  Güterangebotsqualität : Outport  Port=7
  Arbeitslosenquote : Outport  Port=8
  Güterkonsum Ausland : Outport  Port=9
  Kreditbedarf Ausland : Outport  Port=10
  wires:
  Arbeitslohn/1 -> MATLAB Function/7(Arbeitslohn)
  Erwerbsfähige/1 -> MATLAB Function/1(Erwerbsfaehige)
  Arbeitsplätze Dienstleistungen/1 -> MATLAB Function/2(ArbeitsplaetzeDienstleistungen)
  Güterangebot Inland/1 -> MATLAB Function/6(GueterAngebotInland)
  Güterpreis Inland/1 -> MATLAB Function/8(GueterpreisInland)
  MATLAB Function/1(GueterkonsumInland) -> Güterkonsum Inland/1
  MATLAB Function/2(FinanzierungArbeitslosigkeit) -> Finanzbedarf Arbeitslosigkeit/1
  MATLAB Function/4(KreditbedarfInland) -> Kreditbedarf Inland/1
  MATLAB Function/5(ArbeiterUnternehmen) -> Arbeiter Unternehmen/1
  MATLAB Function/3(Spareinlagen) -> Spareinlagen/1
  Neue Kreditvergabe Inland/1 -> MATLAB Function/4(NeueKreditvergabeInland)
  Arbeitsplätze Unternehmen/1 -> MATLAB Function/3(ArbeitsplaetzeUnternehmen)
  MATLAB Function/6(GueterVorratHaushalte) -> Gütervorrat der Haushalte/1
  MATLAB Function/7(GueterangebotsqualitaetOut) -> Güterangebotsqualität/1
  Kreditrückzahlung Ausland/1 -> MATLAB Function/5(KreditrueckzahlungInland)
  MATLAB Function/8(Arbeitslosenquote) -> Arbeitslosenquote/1
  MATLAB Function/9(GueterkonsumAusland) -> Güterkonsum Ausland/1
  MATLAB Function/10(KreditbedarfAusland) -> Kreditbedarf Ausland/1
  Güterpreis Ausland/1 -> MATLAB Function/9(GueterpreisAusland)
  Neue Kreditvergabe Ausland/1 -> MATLAB Function/10(NeueKreditvergabeAusland)
  Kreditrückzahlung Inland/1 -> MATLAB Function/11(KreditrueckzahlungAusland)
  Güterangebot Ausland/1 -> MATLAB Function/12(GueterAngebotAusland)
  Kreditzinssatz Inland/1 -> MATLAB Function/13(KreditZinssatzInland)
  Kreditzinssatz Ausland/1 -> MATLAB Function/14(KreditZinssatzAusland)
